simulink model "DIP"  (R2016b)
settings: Solver=VariableStepAuto  StartTime=0.0  StopTime=5  RelTol=1e-3
libraries: simulink x1
settings Model: Creator=aborowczyk  LastModifiedBy=aborowczyk

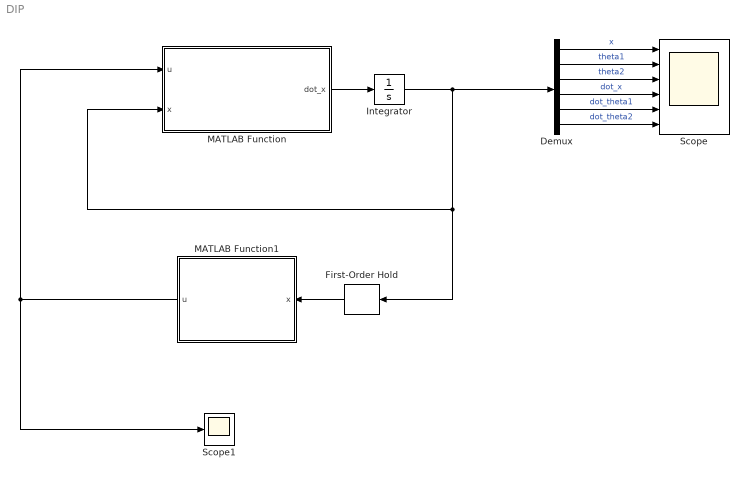
== system DIP ==
  Demux : Demux  Outputs=6
  First-Order Hold : simulink/Discrete/First-Order Hold  DisableCoverage=on  Ts=0.01
  Integrator : Integrator  InitialCondition=[0 deg2rad(1) 0 0 0 0]
  MATLAB Function : MATLAB Function  TreatAsAtomicUnit=on
  MATLAB Function1 : MATLAB Function  TreatAsAtomicUnit=on
  Scope : Scope  NumInputPorts=6
  Scope1 : Scope
  wires:
  MATLAB Function/1(dot_x) -> Integrator/1
  Integrator/1 -> MATLAB Function/2(x), First-Order Hold/1, Demux/1
  Demux/1 -> Scope/1  "x"
  Demux/2 -> Scope/2  "theta1"
  Demux/3 -> Scope/3  "theta2"
  Demux/4 -> Scope/4  "dot_x"
  Demux/5 -> Scope/5  "dot_theta1"
  Demux/6 -> Scope/6  "dot_theta2"
  First-Order Hold/1 -> MATLAB Function1/1(x)
  MATLAB Function1/1(u) -> Scope1/1, MATLAB Function/1(u)

== matlab function DIP/MATLAB Function1 ==
  data: x input; u output
function u  = SDRE_simulink(x)

u = 0;

D = zeros(3);
C = zeros(3);
G = zeros(3);


coder.extrinsic('dare');

% System parameters

m0 = 1.5;  % kg
m1 = 0.5;  % kg
m2 = 0.75; % kg
L1 = 0.5;  % m
L2 = 0.75; % m

Q  = diag([5 50 50 20 700 700]);
R  = 1;

g = 9.81;

% Compupted coefficients

d1 = m0 + m1 + m2;
d2 = (0.5 * m1 + m2) * L1;
d3 = 0.5 * m2 * L2;
d4 = (1/3 * m1 + m2) * L1^2;
d5 = 0.5 * m2 * L1 * L2;
d6 = 1/3 * m2 * L2^2;
f1 = (0.5 * m1 + m2) * L1 * g;
f2 = 0.5 * m2 * L2 * g;

% System dynamics

theta1      = x(2);
theta2      = x(3);
dot_theta1  = x(5);
dot_theta2  = x(6);

D = [d1,              d2*cos(theta1),         d3*cos(theta2);
    d2*cos(theta1),  d4,                     d5*cos(theta1-theta2);
    d3*cos(theta2),  d5*cos(theta1-theta2)   d6];

C = [0, -d2*sin(theta1)*dot_theta1,        -d3*sin(theta2)*dot_theta2;
    0,  0,                                 d5*sin(theta1-theta2)*dot_theta2;
    0  -d5*sin(theta1-theta2)*dot_theta1,  0];

H = [1 0 0]';

% SDRE controler
if 0
    if(deg2rad(0.0001) < abs(theta1))
        G(2,2) = -f1 * sin(theta1)/theta1;
    end
    
    if(deg2rad(0.0001) < abs(theta2))
        G(3,3) = -f2 * sin(theta2)/theta2;
    end
else
    %LQR
    G = diag([0, -f1*cos(theta1), -f2*cos(theta2)]);

end

A = [ zeros(3), eye(3);
    -D\G,  -D\C];

B = [zeros(3,1);
    D\H];

ts = 0.01; % s

AA = expm(A*ts);
BB = B*ts;

% [P,~,~] = care(A,B,Q,R);

[P,~,K] = dare(AA,BB,Q,R);

u = -1*K*x;

== matlab function DIP/MATLAB Function ==
  data: u input; x input; dot_x output
function dot_x  = SystemDerivatives_simulink(u, x)

% System parameters

m0 = 1.5;  % kg
m1 = 0.5;  % kg
m2 = 0.75; % kg
L1 = 0.5;  % m
L2 = 0.75; % m

drag1 = 0.005; % N m s
drag2 = 0.005; % N m s


g = 9.81;

% Compupted coefficients

d1 = m0 + m1 + m2;
d2 = (0.5 * m1 + m2) * L1;
d3 = 0.5 * m2 * L2;
d4 = (1/3 * m1 + m2) * L1^2;
d5 = 0.5 * m2 * L1 * L2;
d6 = 1/3 * m2 * L2^2;
f1 = (0.5 * m1 + m2) * L1 * g;
f2 = 0.5 * m2 * L2 * g;

% System dynamics

theta1      = x(2);
theta2      = x(3);
dot_theta1  = x(5);
dot_theta2  = x(6);

D = [d1,              d2*cos(theta1),         d3*cos(theta2);
     d2*cos(theta1),  d4,                     d5*cos(theta1-theta2);
     d3*cos(theta2),  d5*cos(theta1-theta2)   d6];
 
C = [0, -d2*sin(theta1)*dot_theta1,        -d3*sin(theta2)*dot_theta2;
     0,  0,                                 d5*sin(theta1-theta2)*dot_theta2;
     0  -d5*sin(theta1-theta2)*dot_theta1,  0];
 
G = [0, -f1*sin(theta1), -f2*sin(theta2)]';
 
H = [1 0 0]';

F = [0 -drag1*dot_theta1+drag2*(dot_theta2-dot_theta1) drag2*(dot_theta1-dot_theta2)]';
 
 matrix_1 = [zeros(3), eye(3);
             zeros(3), -D\C];
 matrix_2 = [zeros(3,1); -D\G];
 
 matrix_3 = [zeros(3,1); D\H];
 
 matrix_4 = [zeros(3,1); D\F];
 
dot_x = matrix_1 * x + matrix_2 + matrix_3 * u + matrix_4;
